simulink model "pendulum_model_time_discrete"  (R2022b)
settings: Solver=VariableStepAuto  StartTime=0.0  StopTime=20  RelTol=1e-3
InitFcn:
  | % LRS TU KL %
  | % By Alen Turnwald %
  | % 09.01.2017 %
  | clc
  | close
  | 
  | %% g_q
  | g_q = [1;0];
  | 
  | 
  | if ~exist('mp','var')||~exist('mc','var')||~exist('L','var')||~exist('g','var')||~exist('d1','var')||~exist('d2','var')
  | % Model Paramter
  |     warning(['(Some) Model Parameter are not defined!' ,10, '****  Setting the predefined parameter  ****'])
  |     N = 2;
  |     mc = 1.5;
  |     mp = 0.5;
  |     g = 9.82;
  |     L = 1;
  | % Damping factors
  |     d1 = 1e-2;
  |     d2 = 1e-2;
  | end
  | 
  | if ~exist('x_0','var')
  | % Initial state
  |     warning(['(Initial state "x_0" not defined or wrongly named!' ,10, '****  Setting x_0 = [0.1; 10 deg; 0; 0]  ****'])
  |     x_0 = zeros(4,1);
  |     x_0(1) = 0.1;
  |     x_0(2) = 10*pi/180;
  | end
  | 
  | if ~exist('K_lqr','var')||~exist('Kd_lqr','var')
  |     warning(['(No controller found!' ,10, '****   Applying a predefined controller  ****'])
  |     K_lqr = [-14.1421  171.8846  -25.2787   54.7535];
  | end
StopFcn:
  | %% load data
  | 
  | load output
  | 
  | %% Read data
  | q1 = out.Data(:,1);
  | q2 = out.Data(:,2)*180/pi;
  | x_ref = out.Data(:,5);
  | t = out.Time;
  | 
  | 
  | %% Plot
  | % close all
  | figure(2)
  | clf
  | h(1) = subplot(2,1,1);
  | plot(t,q1,'b','LineWidth',2); grid on
  | 
  | hold on
  | plot(t,x_ref,'r--')
  | hold off
  | ylabel('q_1 [m]')
  | legend('q_1','q_1 ref')
  | 
  | h(2) = subplot(2,1,2);
  | plot(t,q2,'b','LineWidth',2); grid on
  | hold on
  | plot(t,zeros(1,length(t)),'r--')
  | hold off
  | ylabel('q_2 [°]')
  | legend('q_2','q_2 ref')
  | 
  | xlabel('t [s]')
  | 
  | linkaxes(h,'x')
undefined symbols (not defined in the file or in its folder): A, Ad, B, Bd, C, Cd, K_d, Ob, Ts, x0
settings Model: Creator=Jake  LastModifiedBy=Jake

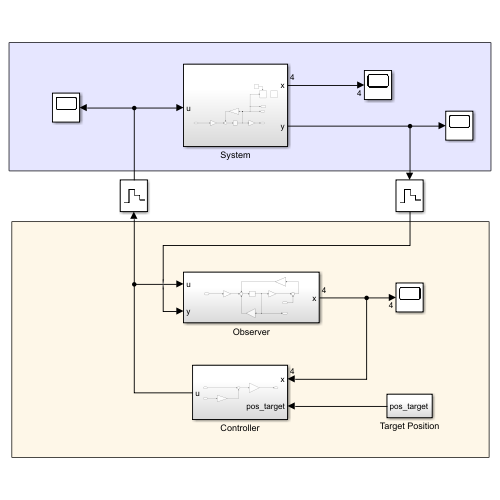
[thumbnail: Simulink's stored preview of the top-level diagram]
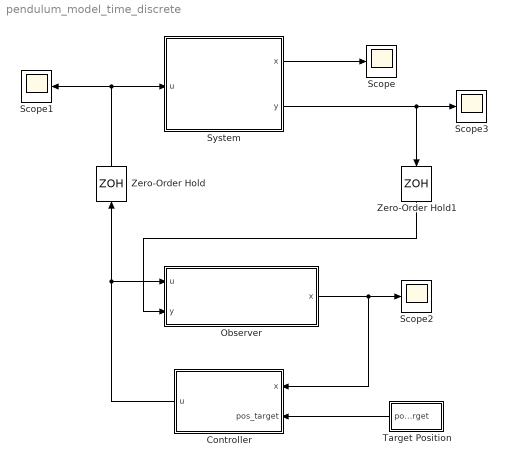
== system pendulum_model_time_discrete ==
  Controller : Subsystem
  Observer : Subsystem
  Scope{,1..3} (4 alike) : Scope
  System : Subsystem
  Target Position : Subsystem
  Zero-Order Hold : ZeroOrderHold  SampleTime=Ts
  Zero-Order Hold1 : ZeroOrderHold  SampleTime=Ts
  wires:
  System/2(y) -> Scope3/1, Zero-Order Hold1/1
  System/1(x) -> Scope/1
  Controller/1(u) -> Zero-Order Hold/1, Observer/1(u)
  Target Position/1(pos_target) -> Controller/2(pos_target)
  Zero-Order Hold/1 -> Scope1/1, System/1(u)
  Zero-Order Hold1/1 -> Observer/2(y)
  Observer/1(x) -> Scope2/1, Controller/1(x)

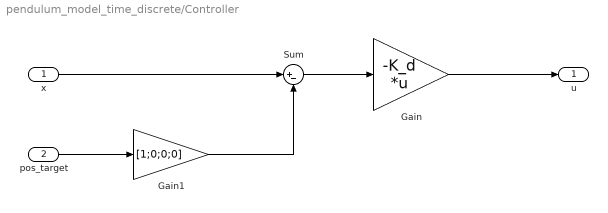
== system pendulum_model_time_discrete/Controller ==
  x : Inport
  pos_target : Inport  Port=2
  Gain : Gain  Gain=-K_d  Multiplication=Matrix(K*u)
  Gain1 : Gain  Gain=[1;0;0;0]
  Sum : Sum  Inputs=|+-
  u : Outport
  wires:
  Gain/1 -> u/1
  Sum/1 -> Gain/1
  x/1 -> Sum/1
  pos_target/1 -> Gain1/1
  Gain1/1 -> Sum/2

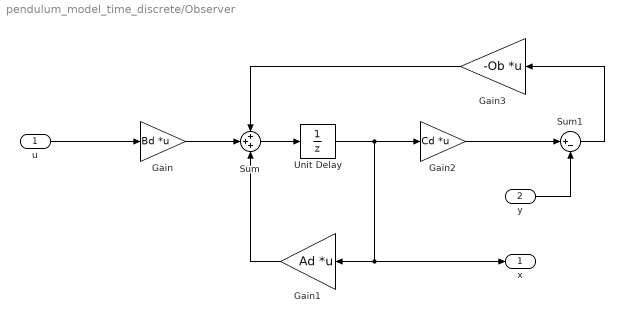
== system pendulum_model_time_discrete/Observer ==
  u : Inport
  y : Inport  Port=2
  Gain : Gain  Gain=Bd  Multiplication=Matrix(K*u)
  Gain1 : Gain  Gain=Ad  Multiplication=Matrix(K*u)
  Gain2 : Gain  Gain=Cd  Multiplication=Matrix(K*u)
  Gain3 : Gain  Gain=-Ob  Multiplication=Matrix(K*u)
  Sum : Sum  Inputs=+++
  Sum1 : Sum  Inputs=|+-
  Unit Delay : UnitDelay  InitialCondition=x0*0  SampleTime=-1  HasFrameUpgradeWarning=on
  x : Outport
  wires:
  Sum/1 -> Unit Delay/1
  Unit Delay/1 -> Gain2/1, Gain1/1, x/1
  u/1 -> Gain/1
  y/1 -> Sum1/2
  Gain2/1 -> Sum1/1
  Sum1/1 -> Gain3/1
  Gain/1 -> Sum/2
  Gain1/1 -> Sum/3
  Gain3/1 -> Sum/1

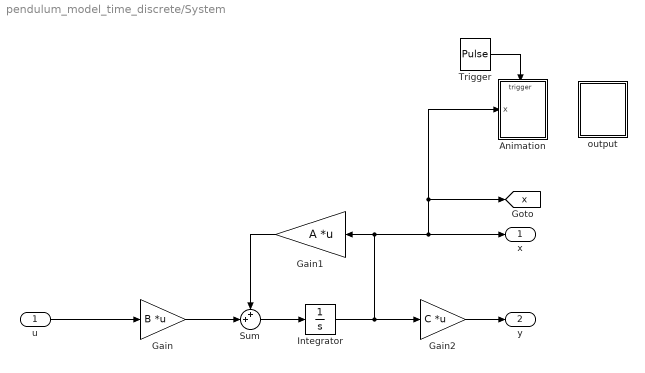
== system pendulum_model_time_discrete/System ==
  u : Inport
  Animation : Subsystem
  Gain : Gain  Gain=B  Multiplication=Matrix(K*u)
  Gain1 : Gain  Gain=A  Multiplication=Matrix(K*u)
  Gain2 : Gain  Gain=C  Multiplication=Matrix(K*u)
  Integrator : Integrator  InitialCondition=x0
  Sum : Sum  Inputs=++|
  Trigger : DiscretePulseGenerator  PulseType=Time based  Period=0.1  PulseWidth=50
  output : Subsystem
  x : Outport
  y : Outport  Port=2
  tag scope: x=global
  wires:
  u/1 -> Gain/1
  Sum/1 -> Integrator/1
  Gain2/1 -> y/1
  Gain1/1 -> Sum/1
  Gain/1 -> Sum/2
  Integrator/1 -> [x], Animation/1(x), x/1, Gain1/1, Gain2/1
  Trigger/1 -> Animation/Trigger

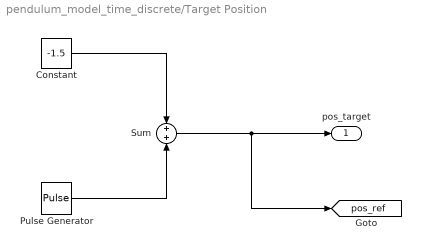
== system pendulum_model_time_discrete/Target Position ==
  Constant : Constant  Value=-1.5
  Pulse Generator : DiscretePulseGenerator  PulseType=Time based  Amplitude=3  Period=20  PulseWidth=50
  Sum : Sum
  pos_target : Outport  VectorParamsAs1DForOutWhenUnconnected=off
  tag scope: pos_ref=global
  wires:
  Sum/1 -> [pos_ref], pos_target/1
  Pulse Generator/1 -> Sum/2
  Constant/1 -> Sum/1

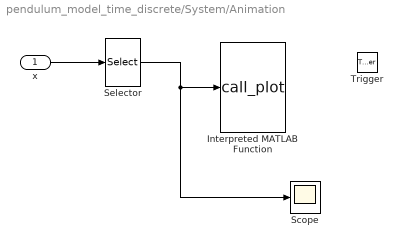
== system pendulum_model_time_discrete/System/Animation ==
  x : Inport
  Trigger : TriggerPort  VariantControl=(inherit)  PortDimensions=1
  Interpreted MATLAB Function : MATLABFcn  MATLABFcn=call_plot  OutputDimensions=0
  Scope : Scope
  Selector : Selector  InputPortWidth=4  IndexOptions=Index vector (dialog)  Indices=[1:2]  OutputSizes=1
  wires:
  x/1 -> Selector/1
  Selector/1 -> Scope/1, Interpreted MATLAB Function/1

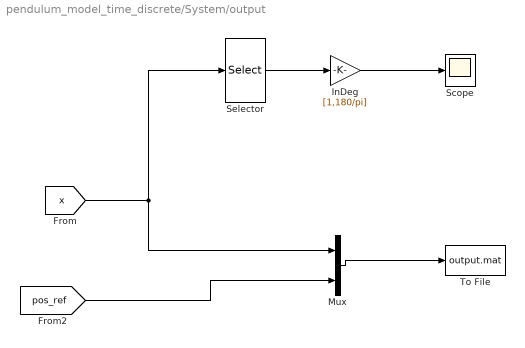
== system pendulum_model_time_discrete/System/output ==
  InDeg : Gain  Gain=[1,180/pi]
  Mux : Mux  Inputs=2
  Scope : Scope
  Selector : Selector  InputPortWidth=4  IndexOptions=Index vector (dialog)  Indices=[1:2]  OutputSizes=1
  To File : ToFile  Filename=output.mat  MatrixName=out  SaveFormat=Timeseries
  wires:
  [x] -> Mux/1, Selector/1
  InDeg/1 -> Scope/1
  Selector/1 -> InDeg/1
  Mux/1 -> To File/1
  [pos_ref] -> Mux/2
